simulink model "fft_direct"  (R2012b)
settings: Solver=ode45  StartTime=0.0  StopTime=199  RelTol=1e-3
libraries: xbsIndex_r4 x2893
(part 1 of 15)
settings Model: Creator=sgowda  LastModifiedBy=sgowda

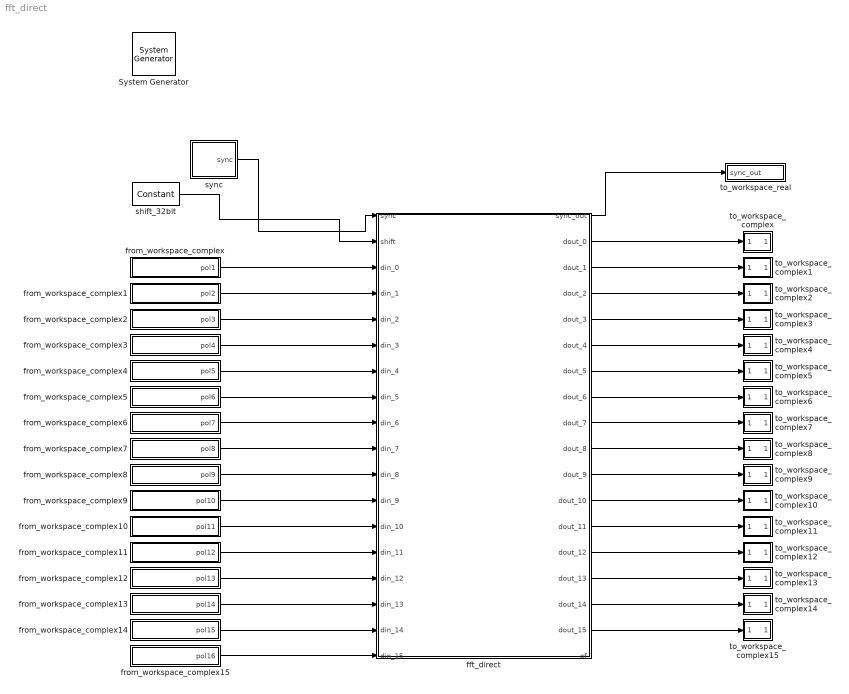
== system fft_direct ==
  " System Generator" : xbsIndex_r4/ System Generator  Tag=genX  xilinxfamily=Kintex7  part=xc7k325t  speed=-3  package=fbg676  synthesis_tool=XST  clock_wrapper=Clock Enables  directory=./netlist  proj_type=Project Navigator  Synth_file=XST Defaults  Impl_file=ISE Defaults  testbench=off  simulink_period=1  sysclk_period=10  dcm_input_clock_period=10  incr_netlist=off  trim_vbits=Everywhere in SubSystem  dbl_ovrd=According to Block Masks  core_generation=According to Block Masks  run_coregen=off  deprecated_control=off  eval_field=0  block_type=sysgen
  fft_direct : Subsystem
  from_workspace_complex : Subsystem  mask{var_name=pol1, n_bits=18, bin_pt=17, quantization=Truncate, overflow=Wrap, arith_type=Signed  (2's comp)}
      mask prompts: var_name "Workspace variable name"; n_bits "# of bits"; bin_pt "Binary Point"; arith_type "Arithmetic type"
      mask init:
      | config.source = str2func('mat_input_data_cplx_init_xblock');
      | config.toplevel = gcb();
      | xBlock(config, {config.toplevel, 'var_name', var_name, ...
      |     'n_bits', n_bits, 'bin_pt', bin_pt, 'quantization', quantization, ...
      |     'overflow', overflow, 'arith_type', arith_type});
      mask TypeOptions quantization: Truncate | Round  (unbiased: +/- Inf) | Round  (unbiased: Even Values)
      mask TypeOptions overflow: Wrap | Saturate | Flag as error
      mask TypeOptions arith_type: Signed  (2's comp) | Boolean | Unsigned
  from_workspace_complex1 : Subsystem  mask{var_name=pol2, n_bits=18, bin_pt=17, quantization=Truncate, overflow=Wrap, arith_type=Signed  (2's comp)}
      mask prompts: var_name "Workspace variable name"; n_bits "# of bits"; bin_pt "Binary Point"; arith_type "Arithmetic type"
      mask init: same as fft_direct/from_workspace_complex
      mask TypeOptions quantization: Truncate | Round  (unbiased: +/- Inf) | Round  (unbiased: Even Values)
      mask TypeOptions overflow: Wrap | Saturate | Flag as error
      mask TypeOptions arith_type: Signed  (2's comp) | Boolean | Unsigned
  from_workspace_complex10 : Subsystem  mask{var_name=pol11, n_bits=18, bin_pt=17, quantization=Truncate, overflow=Wrap, arith_type=Signed  (2's comp)}
      mask prompts: var_name "Workspace variable name"; n_bits "# of bits"; bin_pt "Binary Point"; arith_type "Arithmetic type"
      mask init: same as fft_direct/from_workspace_complex
      mask TypeOptions quantization: Truncate | Round  (unbiased: +/- Inf) | Round  (unbiased: Even Values)
      mask TypeOptions overflow: Wrap | Saturate | Flag as error
      mask TypeOptions arith_type: Signed  (2's comp) | Boolean | Unsigned
  from_workspace_complex11 : Subsystem  mask{var_name=pol12, n_bits=18, bin_pt=17, quantization=Truncate, overflow=Wrap, arith_type=Signed  (2's comp)}
      mask prompts: var_name "Workspace variable name"; n_bits "# of bits"; bin_pt "Binary Point"; arith_type "Arithmetic type"
      mask init: same as fft_direct/from_workspace_complex
      mask TypeOptions quantization: Truncate | Round  (unbiased: +/- Inf) | Round  (unbiased: Even Values)
      mask TypeOptions overflow: Wrap | Saturate | Flag as error
      mask TypeOptions arith_type: Signed  (2's comp) | Boolean | Unsigned
  from_workspace_complex12 : Subsystem  mask{var_name=pol13, n_bits=18, bin_pt=17, quantization=Truncate, overflow=Wrap, arith_type=Signed  (2's comp)}
      mask prompts: var_name "Workspace variable name"; n_bits "# of bits"; bin_pt "Binary Point"; arith_type "Arithmetic type"
      mask init: same as fft_direct/from_workspace_complex
      mask TypeOptions quantization: Truncate | Round  (unbiased: +/- Inf) | Round  (unbiased: Even Values)
      mask TypeOptions overflow: Wrap | Saturate | Flag as error
      mask TypeOptions arith_type: Signed  (2's comp) | Boolean | Unsigned
  from_workspace_complex13 : Subsystem  mask{var_name=pol14, n_bits=18, bin_pt=17, quantization=Truncate, overflow=Wrap, arith_type=Signed  (2's comp)}
      mask prompts: var_name "Workspace variable name"; n_bits "# of bits"; bin_pt "Binary Point"; arith_type "Arithmetic type"
      mask init: same as fft_direct/from_workspace_complex
      mask TypeOptions quantization: Truncate | Round  (unbiased: +/- Inf) | Round  (unbiased: Even Values)
      mask TypeOptions overflow: Wrap | Saturate | Flag as error
      mask TypeOptions arith_type: Signed  (2's comp) | Boolean | Unsigned
  from_workspace_complex14 : Subsystem  mask{var_name=pol15, n_bits=18, bin_pt=17, quantization=Truncate, overflow=Wrap, arith_type=Signed  (2's comp)}
      mask prompts: var_name "Workspace variable name"; n_bits "# of bits"; bin_pt "Binary Point"; arith_type "Arithmetic type"
      mask init: same as fft_direct/from_workspace_complex
      mask TypeOptions quantization: Truncate | Round  (unbiased: +/- Inf) | Round  (unbiased: Even Values)
      mask TypeOptions overflow: Wrap | Saturate | Flag as error
      mask TypeOptions arith_type: Signed  (2's comp) | Boolean | Unsigned
  from_workspace_complex15 : Subsystem  mask{var_name=pol16, n_bits=18, bin_pt=17, quantization=Truncate, overflow=Wrap, arith_type=Signed  (2's comp)}
      mask prompts: var_name "Workspace variable name"; n_bits "# of bits"; bin_pt "Binary Point"; arith_type "Arithmetic type"
      mask init: same as fft_direct/from_workspace_complex
      mask TypeOptions quantization: Truncate | Round  (unbiased: +/- Inf) | Round  (unbiased: Even Values)
      mask TypeOptions overflow: Wrap | Saturate | Flag as error
      mask TypeOptions arith_type: Signed  (2's comp) | Boolean | Unsigned
  from_workspace_complex2 : Subsystem  mask{var_name=pol3, n_bits=18, bin_pt=17, quantization=Truncate, overflow=Wrap, arith_type=Signed  (2's comp)}
      mask prompts: var_name "Workspace variable name"; n_bits "# of bits"; bin_pt "Binary Point"; arith_type "Arithmetic type"
      mask init: same as fft_direct/from_workspace_complex
      mask TypeOptions quantization: Truncate | Round  (unbiased: +/- Inf) | Round  (unbiased: Even Values)
      mask TypeOptions overflow: Wrap | Saturate | Flag as error
      mask TypeOptions arith_type: Signed  (2's comp) | Boolean | Unsigned
  from_workspace_complex3 : Subsystem  mask{var_name=pol4, n_bits=18, bin_pt=17, quantization=Truncate, overflow=Wrap, arith_type=Signed  (2's comp)}
      mask prompts: var_name "Workspace variable name"; n_bits "# of bits"; bin_pt "Binary Point"; arith_type "Arithmetic type"
      mask init: same as fft_direct/from_workspace_complex
      mask TypeOptions quantization: Truncate | Round  (unbiased: +/- Inf) | Round  (unbiased: Even Values)
      mask TypeOptions overflow: Wrap | Saturate | Flag as error
      mask TypeOptions arith_type: Signed  (2's comp) | Boolean | Unsigned
  from_workspace_complex4 : Subsystem  mask{var_name=pol5, n_bits=18, bin_pt=17, quantization=Truncate, overflow=Wrap, arith_type=Signed  (2's comp)}
      mask prompts: var_name "Workspace variable name"; n_bits "# of bits"; bin_pt "Binary Point"; arith_type "Arithmetic type"
      mask init: same as fft_direct/from_workspace_complex
      mask TypeOptions quantization: Truncate | Round  (unbiased: +/- Inf) | Round  (unbiased: Even Values)
      mask TypeOptions overflow: Wrap | Saturate | Flag as error
      mask TypeOptions arith_type: Signed  (2's comp) | Boolean | Unsigned
  from_workspace_complex5 : Subsystem  mask{var_name=pol6, n_bits=18, bin_pt=17, quantization=Truncate, overflow=Wrap, arith_type=Signed  (2's comp)}
      mask prompts: var_name "Workspace variable name"; n_bits "# of bits"; bin_pt "Binary Point"; arith_type "Arithmetic type"
      mask init: same as fft_direct/from_workspace_complex
      mask TypeOptions quantization: Truncate | Round  (unbiased: +/- Inf) | Round  (unbiased: Even Values)
      mask TypeOptions overflow: Wrap | Saturate | Flag as error
      mask TypeOptions arith_type: Signed  (2's comp) | Boolean | Unsigned
  from_workspace_complex6 : Subsystem  mask{var_name=pol7, n_bits=18, bin_pt=17, quantization=Truncate, overflow=Wrap, arith_type=Signed  (2's comp)}
      mask prompts: var_name "Workspace variable name"; n_bits "# of bits"; bin_pt "Binary Point"; arith_type "Arithmetic type"
      mask init: same as fft_direct/from_workspace_complex
      mask TypeOptions quantization: Truncate | Round  (unbiased: +/- Inf) | Round  (unbiased: Even Values)
      mask TypeOptions overflow: Wrap | Saturate | Flag as error
      mask TypeOptions arith_type: Signed  (2's comp) | Boolean | Unsigned
  from_workspace_complex7 : Subsystem  mask{var_name=pol8, n_bits=18, bin_pt=17, quantization=Truncate, overflow=Wrap, arith_type=Signed  (2's comp)}
      mask prompts: var_name "Workspace variable name"; n_bits "# of bits"; bin_pt "Binary Point"; arith_type "Arithmetic type"
      mask init: same as fft_direct/from_workspace_complex
      mask TypeOptions quantization: Truncate | Round  (unbiased: +/- Inf) | Round  (unbiased: Even Values)
      mask TypeOptions overflow: Wrap | Saturate | Flag as error
      mask TypeOptions arith_type: Signed  (2's comp) | Boolean | Unsigned
  from_workspace_complex8 : Subsystem  mask{var_name=pol9, n_bits=18, bin_pt=17, quantization=Truncate, overflow=Wrap, arith_type=Signed  (2's comp)}
      mask prompts: var_name "Workspace variable name"; n_bits "# of bits"; bin_pt "Binary Point"; arith_type "Arithmetic type"
      mask init: same as fft_direct/from_workspace_complex
      mask TypeOptions quantization: Truncate | Round  (unbiased: +/- Inf) | Round  (unbiased: Even Values)
      mask TypeOptions overflow: Wrap | Saturate | Flag as error
      mask TypeOptions arith_type: Signed  (2's comp) | Boolean | Unsigned
  from_workspace_complex9 : Subsystem  mask{var_name=pol10, n_bits=18, bin_pt=17, quantization=Truncate, overflow=Wrap, arith_type=Signed  (2's comp)}
      mask prompts: var_name "Workspace variable name"; n_bits "# of bits"; bin_pt "Binary Point"; arith_type "Arithmetic type"
      mask init: same as fft_direct/from_workspace_complex
      mask TypeOptions quantization: Truncate | Round  (unbiased: +/- Inf) | Round  (unbiased: Even Values)
      mask TypeOptions overflow: Wrap | Saturate | Flag as error
      mask TypeOptions arith_type: Signed  (2's comp) | Boolean | Unsigned
  shift_32bit : xbsIndex_r4/Constant  const=0  gui_display_data_type=Fixed-point  arith_type=Signed (2's comp)  n_bits=32  bin_pt=0  preci_type=Single  exp_width=8  frac_width=24  explicit_period=on  period=1  equ=P=C  opselect=C  inp2=PCIN>>17  opr=+  inp1=P  carry=CIN  dbl_ovrd=off  block_type=constant
  sync : Subsystem
  to_workspace_complex : Subsystem  mask{var_name=out1, n_bits=18, bin_pt=17}
      mask prompts: var_name "Workspace variable name"; n_bits "# of bits"; bin_pt "Binary Point"
      mask init:
      | config.source = str2func('mat_output_data_cplx_init_xblock');
      | config.toplevel = gcb();
      | xBlock(config, {config.toplevel, 'var_name', var_name, ...
      |     'n_bits', n_bits, 'bin_pt', bin_pt});
  to_workspace_complex1 : Subsystem  mask{var_name=out2, n_bits=18, bin_pt=17}
      mask prompts: var_name "Workspace variable name"; n_bits "# of bits"; bin_pt "Binary Point"
      mask init:
      | config.source = str2func('mat_output_data_cplx_init_xblock');
      | config.toplevel = gcb();
      | xBlock(config, {config.toplevel, 'var_name', var_name, ...
      |     'n_bits', n_bits, 'bin_pt', bin_pt});
  to_workspace_complex10 : Subsystem  mask{var_name=out11, n_bits=18, bin_pt=17}
      mask prompts: var_name "Workspace variable name"; n_bits "# of bits"; bin_pt "Binary Point"
      mask init:
      | config.source = str2func('mat_output_data_cplx_init_xblock');
      | config.toplevel = gcb();
      | xBlock(config, {config.toplevel, 'var_name', var_name, ...
      |     'n_bits', n_bits, 'bin_pt', bin_pt});
  to_workspace_complex11 : Subsystem  mask{var_name=out12, n_bits=18, bin_pt=17}
      mask prompts: var_name "Workspace variable name"; n_bits "# of bits"; bin_pt "Binary Point"
      mask init:
      | config.source = str2func('mat_output_data_cplx_init_xblock');
      | config.toplevel = gcb();
      | xBlock(config, {config.toplevel, 'var_name', var_name, ...
      |     'n_bits', n_bits, 'bin_pt', bin_pt});
  to_workspace_complex12 : Subsystem  mask{var_name=out13, n_bits=18, bin_pt=17}
      mask prompts: var_name "Workspace variable name"; n_bits "# of bits"; bin_pt "Binary Point"
      mask init:
      | config.source = str2func('mat_output_data_cplx_init_xblock');
      | config.toplevel = gcb();
      | xBlock(config, {config.toplevel, 'var_name', var_name, ...
      |     'n_bits', n_bits, 'bin_pt', bin_pt});
  to_workspace_complex13 : Subsystem  mask{var_name=out14, n_bits=18, bin_pt=17}
      mask prompts: var_name "Workspace variable name"; n_bits "# of bits"; bin_pt "Binary Point"
      mask init:
      | config.source = str2func('mat_output_data_cplx_init_xblock');
      | config.toplevel = gcb();
      | xBlock(config, {config.toplevel, 'var_name', var_name, ...
      |     'n_bits', n_bits, 'bin_pt', bin_pt});
  to_workspace_complex14 : Subsystem  mask{var_name=out15, n_bits=18, bin_pt=17}
      mask prompts: var_name "Workspace variable name"; n_bits "# of bits"; bin_pt "Binary Point"
      mask init:
      | config.source = str2func('mat_output_data_cplx_init_xblock');
      | config.toplevel = gcb();
      | xBlock(config, {config.toplevel, 'var_name', var_name, ...
      |     'n_bits', n_bits, 'bin_pt', bin_pt});
  to_workspace_complex15 : Subsystem  mask{var_name=out16, n_bits=18, bin_pt=17}
      mask prompts: var_name "Workspace variable name"; n_bits "# of bits"; bin_pt "Binary Point"
      mask init:
      | config.source = str2func('mat_output_data_cplx_init_xblock');
      | config.toplevel = gcb();
      | xBlock(config, {config.toplevel, 'var_name', var_name, ...
      |     'n_bits', n_bits, 'bin_pt', bin_pt});
  to_workspace_complex2 : Subsystem  mask{var_name=out3, n_bits=18, bin_pt=17}
      mask prompts: var_name "Workspace variable name"; n_bits "# of bits"; bin_pt "Binary Point"
      mask init:
      | config.source = str2func('mat_output_data_cplx_init_xblock');
      | config.toplevel = gcb();
      | xBlock(config, {config.toplevel, 'var_name', var_name, ...
      |     'n_bits', n_bits, 'bin_pt', bin_pt});
  to_workspace_complex3 : Subsystem  mask{var_name=out4, n_bits=18, bin_pt=17}
      mask prompts: var_name "Workspace variable name"; n_bits "# of bits"; bin_pt "Binary Point"
      mask init:
      | config.source = str2func('mat_output_data_cplx_init_xblock');
      | config.toplevel = gcb();
      | xBlock(config, {config.toplevel, 'var_name', var_name, ...
      |     'n_bits', n_bits, 'bin_pt', bin_pt});
  to_workspace_complex4 : Subsystem  mask{var_name=out5, n_bits=18, bin_pt=17}
      mask prompts: var_name "Workspace variable name"; n_bits "# of bits"; bin_pt "Binary Point"
      mask init:
      | config.source = str2func('mat_output_data_cplx_init_xblock');
      | config.toplevel = gcb();
      | xBlock(config, {config.toplevel, 'var_name', var_name, ...
      |     'n_bits', n_bits, 'bin_pt', bin_pt});
  to_workspace_complex5 : Subsystem  mask{var_name=out6, n_bits=18, bin_pt=17}
      mask prompts: var_name "Workspace variable name"; n_bits "# of bits"; bin_pt "Binary Point"
      mask init:
      | config.source = str2func('mat_output_data_cplx_init_xblock');
      | config.toplevel = gcb();
      | xBlock(config, {config.toplevel, 'var_name', var_name, ...
      |     'n_bits', n_bits, 'bin_pt', bin_pt});
  to_workspace_complex6 : Subsystem  mask{var_name=out7, n_bits=18, bin_pt=17}
      mask prompts: var_name "Workspace variable name"; n_bits "# of bits"; bin_pt "Binary Point"
      mask init:
      | config.source = str2func('mat_output_data_cplx_init_xblock');
      | config.toplevel = gcb();
      | xBlock(config, {config.toplevel, 'var_name', var_name, ...
      |     'n_bits', n_bits, 'bin_pt', bin_pt});
  to_workspace_complex7 : Subsystem  mask{var_name=out8, n_bits=18, bin_pt=17}
      mask prompts: var_name "Workspace variable name"; n_bits "# of bits"; bin_pt "Binary Point"
      mask init:
      | config.source = str2func('mat_output_data_cplx_init_xblock');
      | config.toplevel = gcb();
      | xBlock(config, {config.toplevel, 'var_name', var_name, ...
      |     'n_bits', n_bits, 'bin_pt', bin_pt});
  to_workspace_complex8 : Subsystem  mask{var_name=out9, n_bits=18, bin_pt=17}
      mask prompts: var_name "Workspace variable name"; n_bits "# of bits"; bin_pt "Binary Point"
      mask init:
      | config.source = str2func('mat_output_data_cplx_init_xblock');
      | config.toplevel = gcb();
      | xBlock(config, {config.toplevel, 'var_name', var_name, ...
      |     'n_bits', n_bits, 'bin_pt', bin_pt});
  to_workspace_complex9 : Subsystem  mask{var_name=out10, n_bits=18, bin_pt=17}
      mask prompts: var_name "Workspace variable name"; n_bits "# of bits"; bin_pt "Binary Point"
      mask init:
      | config.source = str2func('mat_output_data_cplx_init_xblock');
      | config.toplevel = gcb();
      | xBlock(config, {config.toplevel, 'var_name', var_name, ...
      |     'n_bits', n_bits, 'bin_pt', bin_pt});
  to_workspace_real : Subsystem  mask{var_name=sync_out}
      mask prompts: var_name "Workspace variable name"
      mask init:
      | config.source = str2func('mat_output_data_init_xblock');
      | config.toplevel = gcb();
      | xBlock(config, {config.toplevel, 'var_name', var_name});
  wires:
  shift_32bit/1 -> fft_direct/2(shift)
  sync/1(sync) -> fft_direct/1(sync)
  from_workspace_complex/1(pol1) -> fft_direct/3(din_0)
  from_workspace_complex2/1(pol3) -> fft_direct/5(din_2)
  from_workspace_complex3/1(pol4) -> fft_direct/6(din_3)
  fft_direct/1(sync_out) -> to_workspace_real/1(sync_out)
  fft_direct/2(dout_0) -> to_workspace_complex/1(out1)
  fft_direct/3(dout_1) -> to_workspace_complex1/1(out2)
  fft_direct/4(dout_2) -> to_workspace_complex2/1(out3)
  fft_direct/5(dout_3) -> to_workspace_complex3/1(out4)
  from_workspace_complex1/1(pol2) -> fft_direct/4(din_1)
  from_workspace_complex4/1(pol5) -> fft_direct/7(din_4)
  from_workspace_complex5/1(pol6) -> fft_direct/8(din_5)
  from_workspace_complex6/1(pol7) -> fft_direct/9(din_6)
  from_workspace_complex7/1(pol8) -> fft_direct/10(din_7)
  fft_direct/6(dout_4) -> to_workspace_complex4/1(out5)
  fft_direct/7(dout_5) -> to_workspace_complex5/1(out6)
  fft_direct/8(dout_6) -> to_workspace_complex6/1(out7)
  fft_direct/9(dout_7) -> to_workspace_complex7/1(out8)
  from_workspace_complex10/1(pol11) -> fft_direct/13(din_10)
  from_workspace_complex11/1(pol12) -> fft_direct/14(din_11)
  from_workspace_complex13/1(pol14) -> fft_direct/16(din_13)
  from_workspace_complex14/1(pol15) -> fft_direct/17(din_14)
  from_workspace_complex15/1(pol16) -> fft_direct/18(din_15)
  from_workspace_complex12/1(pol13) -> fft_direct/15(din_12)
  from_workspace_complex8/1(pol9) -> fft_direct/11(din_8)
  from_workspace_complex9/1(pol10) -> fft_direct/12(din_9)
  fft_direct/10(dout_8) -> to_workspace_complex8/1(out9)
  fft_direct/11(dout_9) -> to_workspace_complex9/1(out10)
  fft_direct/12(dout_10) -> to_workspace_complex10/1(out11)
  fft_direct/13(dout_11) -> to_workspace_complex11/1(out12)
  fft_direct/14(dout_12) -> to_workspace_complex12/1(out13)
  fft_direct/15(dout_13) -> to_workspace_complex13/1(out14)
  fft_direct/16(dout_14) -> to_workspace_complex14/1(out15)
  fft_direct/17(dout_15) -> to_workspace_complex15/1(out16)

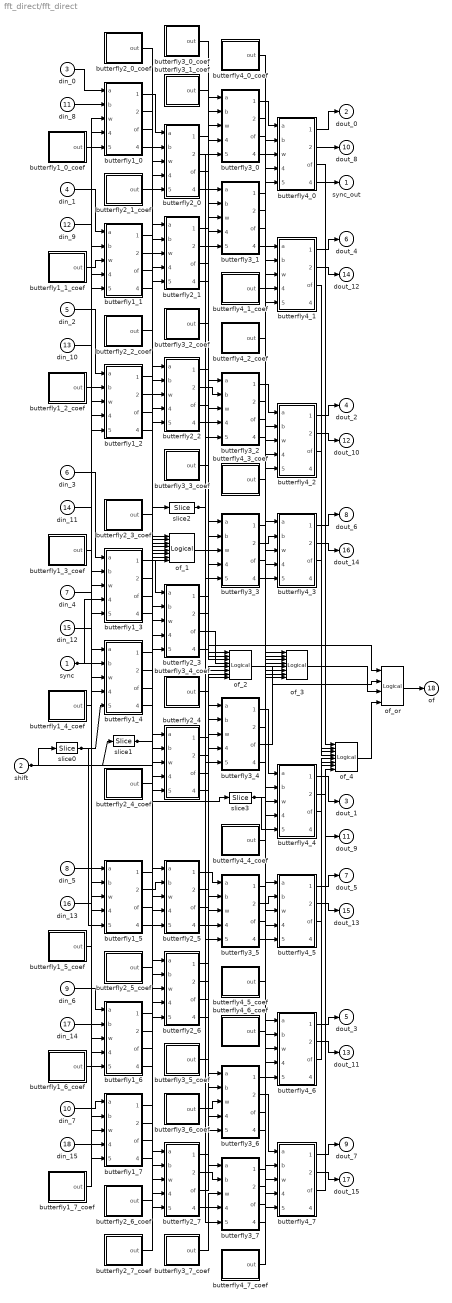
== system fft_direct/fft_direct ==
  sync : Inport
  shift : Inport  Port=2
  din_0 : Inport  Port=3
  din_1 : Inport  Port=4
  din_2 : Inport  Port=5
  din_3 : Inport  Port=6
  din_4 : Inport  Port=7
  din_5 : Inport  Port=8
  din_6 : Inport  Port=9
  din_7 : Inport  Port=10
  din_8 : Inport  Port=11
  din_9 : Inport  Port=12
  din_10 : Inport  Port=13
  din_11 : Inport  Port=14
  din_12 : Inport  Port=15
  din_13 : Inport  Port=16
  din_14 : Inport  Port=17
  din_15 : Inport  Port=18
  butterfly1_0 : Subsystem
      settings: AttributesFormatString=|
      | twiddle_pass_through
      | coeffs in slices
      | Bit growth:0
  butterfly1_0_coef : Subsystem
  butterfly1_1 : Subsystem
      settings: AttributesFormatString=|
      | twiddle_pass_through
      | coeffs in slices
      | Bit growth:0
  butterfly1_1_coef : Subsystem
  butterfly1_2 : Subsystem
      settings: AttributesFormatString=|
      | twiddle_pass_through
      | coeffs in slices
      | Bit growth:0
  butterfly1_2_coef : Subsystem
  butterfly1_3 : Subsystem
      settings: AttributesFormatString=|
      | twiddle_pass_through
      | coeffs in slices
      | Bit growth:0
  butterfly1_3_coef : Subsystem
  butterfly1_4 : Subsystem
      settings: AttributesFormatString=|
      | twiddle_pass_through
      | coeffs in slices
      | Bit growth:0
  butterfly1_4_coef : Subsystem
  butterfly1_5 : Subsystem
      settings: AttributesFormatString=|
      | twiddle_pass_through
      | coeffs in slices
      | Bit growth:0
  butterfly1_5_coef : Subsystem
  butterfly1_6 : Subsystem
      settings: AttributesFormatString=|
      | twiddle_pass_through
      | coeffs in slices
      | Bit growth:0
  butterfly1_6_coef : Subsystem
  butterfly1_7 : Subsystem
      settings: AttributesFormatString=|
      | twiddle_pass_through
      | coeffs in slices
      | Bit growth:0
  butterfly1_7_coef : Subsystem
  butterfly2_0 : Subsystem
      settings: AttributesFormatString=|
      | twiddle_pass_through
      | coeffs in slices
      | Bit growth:0
  butterfly2_0_coef : Subsystem
  butterfly2_1 : Subsystem
      settings: AttributesFormatString=|
      | twiddle_pass_through
      | coeffs in slices
      | Bit growth:0
  butterfly2_1_coef : Subsystem
  butterfly2_2 : Subsystem
      settings: AttributesFormatString=|
      | twiddle_pass_through
      | coeffs in slices
      | Bit growth:0
  butterfly2_2_coef : Subsystem
  butterfly2_3 : Subsystem
      settings: AttributesFormatString=|
      | twiddle_pass_through
      | coeffs in slices
      | Bit growth:0
  butterfly2_3_coef : Subsystem
  butterfly2_4 : Subsystem
      settings: AttributesFormatString=|
      | twiddle_coeff_1
      | coeffs in slices
      | Bit growth:0
  butterfly2_4_coef : Subsystem
  butterfly2_5 : Subsystem
      settings: AttributesFormatString=|
      | twiddle_coeff_1
      | coeffs in slices
      | Bit growth:0
  butterfly2_5_coef : Subsystem
  butterfly2_6 : Subsystem
      settings: AttributesFormatString=|
      | twiddle_coeff_1
      | coeffs in slices
      | Bit growth:0
  butterfly2_6_coef : Subsystem
  butterfly2_7 : Subsystem
      settings: AttributesFormatString=|
      | twiddle_coeff_1
      | coeffs in slices
      | Bit growth:0
  butterfly2_7_coef : Subsystem
  butterfly3_0 : Subsystem
      settings: AttributesFormatString=|
      | twiddle_general_4mult
      | coeffs in slices
      | Bit growth:0
  butterfly3_0_coef : Subsystem
  butterfly3_1 : Subsystem
      settings: AttributesFormatString=|
      | twiddle_general_4mult
      | coeffs in slices
      | Bit growth:0
  butterfly3_1_coef : Subsystem
  butterfly3_2 : Subsystem
      settings: AttributesFormatString=|
      | twiddle_general_4mult
      | coeffs in slices
      | Bit growth:0
  butterfly3_2_coef : Subsystem
  butterfly3_3 : Subsystem
      settings: AttributesFormatString=|
      | twiddle_general_4mult
      | coeffs in slices
      | Bit growth:0
  butterfly3_3_coef : Subsystem
  butterfly3_4 : Subsystem
      settings: AttributesFormatString=|
      | twiddle_general_4mult
      | coeffs in slices
      | Bit growth:0
  butterfly3_4_coef : Subsystem
  butterfly3_5 : Subsystem
      settings: AttributesFormatString=|
      | twiddle_general_4mult
      | coeffs in slices
      | Bit growth:0
  butterfly3_5_coef : Subsystem
  butterfly3_6 : Subsystem
      settings: AttributesFormatString=|
      | twiddle_general_4mult
      | coeffs in slices
      | Bit growth:0
  butterfly3_6_coef : Subsystem
  butterfly3_7 : Subsystem
      settings: AttributesFormatString=|
      | twiddle_general_4mult
      | coeffs in slices
      | Bit growth:0
  butterfly3_7_coef : Subsystem
  butterfly4_0 : Subsystem
      settings: AttributesFormatString=|
      | twiddle_general_4mult
      | coeffs in slices
      | Bit growth:0
  butterfly4_0_coef : Subsystem
  butterfly4_1 : Subsystem
      settings: AttributesFormatString=|
      | twiddle_general_4mult
      | coeffs in slices
      | Bit growth:0
  butterfly4_1_coef : Subsystem
  butterfly4_2 : Subsystem
      settings: AttributesFormatString=|
      | twiddle_general_4mult
      | coeffs in slices
      | Bit growth:0
  butterfly4_2_coef : Subsystem
  butterfly4_3 : Subsystem
      settings: AttributesFormatString=|
      | twiddle_general_4mult
      | coeffs in slices
      | Bit growth:0
  butterfly4_3_coef : Subsystem
  butterfly4_4 : Subsystem
      settings: AttributesFormatString=|
      | twiddle_general_4mult
      | coeffs in slices
      | Bit growth:0
  butterfly4_4_coef : Subsystem
  butterfly4_5 : Subsystem
      settings: AttributesFormatString=|
      | twiddle_general_4mult
      | coeffs in slices
      | Bit growth:0
  butterfly4_5_coef : Subsystem
  butterfly4_6 : Subsystem
      settings: AttributesFormatString=|
      | twiddle_general_4mult
      | coeffs in slices
      | Bit growth:0
  butterfly4_6_coef : Subsystem
  butterfly4_7 : Subsystem
      settings: AttributesFormatString=|
      | twiddle_general_4mult
      | coeffs in slices
      | Bit growth:0
  butterfly4_7_coef : Subsystem
  of_{1..4} (4 alike) : xbsIndex_r4/Logical  logical_function=OR  inputs=8  en=off  latency=1  precision=Full  arith_type=Unsigned  n_bits=16  bin_pt=0  align_bp=on  dbl_ovrd=off  block_type=logical
  of_or : xbsIndex_r4/Logical  logical_function=OR  inputs=4  en=off  latency=0  precision=Full  arith_type=Unsigned  n_bits=16  bin_pt=0  align_bp=on  dbl_ovrd=off  block_type=logical
  slice0 : xbsIndex_r4/Slice  nbits=1  boolean_output=on  mode=Lower Bit Location + Width  bit1=0  base1=MSB of Input  bit0=0  base0=LSB of Input  dbl_ovrd=off  block_type=slice
  slice1 : xbsIndex_r4/Slice  nbits=1  boolean_output=on  mode=Lower Bit Location + Width  bit1=0  base1=MSB of Input  bit0=1  base0=LSB of Input  dbl_ovrd=off  block_type=slice
  slice2 : xbsIndex_r4/Slice  nbits=1  boolean_output=on  mode=Lower Bit Location + Width  bit1=0  base1=MSB of Input  bit0=2  base0=LSB of Input  dbl_ovrd=off  block_type=slice
  slice3 : xbsIndex_r4/Slice  nbits=1  boolean_output=on  mode=Lower Bit Location + Width  bit1=0  base1=MSB of Input  bit0=3  base0=LSB of Input  dbl_ovrd=off  block_type=slice
  sync_out : Outport
  dout_0 : Outport  Port=2
  dout_1 : Outport  Port=3
  dout_2 : Outport  Port=4
  dout_3 : Outport  Port=5
  dout_4 : Outport  Port=6
  dout_5 : Outport  Port=7
  dout_6 : Outport  Port=8
  dout_7 : Outport  Port=9
  dout_8 : Outport  Port=10
  dout_9 : Outport  Port=11
  dout_10 : Outport  Port=12
  dout_11 : Outport  Port=13
  dout_12 : Outport  Port=14
  dout_13 : Outport  Port=15
  dout_14 : Outport  Port=16
  dout_15 : Outport  Port=17
  of : Outport  Port=18
  wires:
  shift/1 -> slice3/1, slice2/1, slice1/1, slice0/1
  sync/1 -> butterfly1_7/4(sync), butterfly1_6/4(sync), butterfly1_5/4(sync), butterfly1_4/4(sync), butterfly1_3/4(sync), butterfly1_2/4(sync), butterfly1_1/4(sync), butterfly1_0/4(sync)
  slice0/1 -> butterfly1_7/5(shift), butterfly1_6/5(shift), butterfly1_5/5(shift), butterfly1_4/5(shift), butterfly1_3/5(shift), butterfly1_2/5(shift), butterfly1_1/5(shift), butterfly1_0/5(shift)
  slice1/1 -> butterfly2_7/5(shift), butterfly2_6/5(shift), butterfly2_5/5(shift), butterfly2_4/5(shift), butterfly2_3/5(shift), butterfly2_2/5(shift), butterfly2_1/5(shift), butterfly2_0/5(shift)
  slice2/1 -> butterfly3_7/5(shift), butterfly3_6/5(shift), butterfly3_5/5(shift), butterfly3_4/5(shift), butterfly3_3/5(shift), butterfly3_2/5(shift), butterfly3_1/5(shift), butterfly3_0/5(shift)
  slice3/1 -> butterfly4_7/5(shift), butterfly4_6/5(shift), butterfly4_5/5(shift), butterfly4_4/5(shift), butterfly4_3/5(shift), butterfly4_2/5(shift), butterfly4_1/5(shift), butterfly4_0/5(shift)
  butterfly4_7/2(a-bw) -> dout_15/1
  butterfly4_3/2(a-bw) -> dout_14/1
  butterfly4_5/2(a-bw) -> dout_13/1
  butterfly4_1/2(a-bw) -> dout_12/1
  butterfly4_6/2(a-bw) -> dout_11/1
  butterfly4_2/2(a-bw) -> dout_10/1
  butterfly4_4/2(a-bw) -> dout_9/1
  butterfly4_0/2(a-bw) -> dout_8/1
  butterfly4_7/1(a+bw) -> dout_7/1
  butterfly4_3/1(a+bw) -> dout_6/1
  butterfly4_5/1(a+bw) -> dout_5/1
  butterfly4_1/1(a+bw) -> dout_4/1
  butterfly4_6/1(a+bw) -> dout_3/1
  butterfly4_2/1(a+bw) -> dout_2/1
  butterfly4_4/1(a+bw) -> dout_1/1
  butterfly4_0/1(a+bw) -> dout_0/1
  of_or/1 -> of/1
  of_4/1 -> of_or/4
  of_3/1 -> of_or/3
  of_2/1 -> of_or/2
  of_1/1 -> of_or/1
  butterfly4_7/3(of) -> of_4/8
  butterfly4_6/3(of) -> of_4/7
  butterfly4_5/3(of) -> of_4/6
  butterfly4_4/3(of) -> of_4/5
  butterfly4_3/3(of) -> of_4/4
  butterfly4_2/3(of) -> of_4/3
  butterfly4_1/3(of) -> of_4/2
  butterfly4_0/3(of) -> of_4/1
  butterfly3_7/4(sync_out) -> butterfly4_7/4(sync)
  butterfly4_7_coef/1(out) -> butterfly4_7/3(w)
  butterfly3_7/2(a-bw) -> butterfly4_7/2(b)
  butterfly3_6/2(a-bw) -> butterfly4_7/1(a)
  butterfly3_6/4(sync_out) -> butterfly4_6/4(sync)
  butterfly4_6_coef/1(out) -> butterfly4_6/3(w)
  butterfly3_7/1(a+bw) -> butterfly4_6/2(b)
  butterfly3_6/1(a+bw) -> butterfly4_6/1(a)
  butterfly3_5/4(sync_out) -> butterfly4_5/4(sync)
  butterfly4_5_coef/1(out) -> butterfly4_5/3(w)
  butterfly3_5/2(a-bw) -> butterfly4_5/2(b)
  butterfly3_4/2(a-bw) -> butterfly4_5/1(a)
  butterfly3_4/4(sync_out) -> butterfly4_4/4(sync)
  butterfly4_4_coef/1(out) -> butterfly4_4/3(w)
  butterfly3_5/1(a+bw) -> butterfly4_4/2(b)
  butterfly3_4/1(a+bw) -> butterfly4_4/1(a)
  butterfly3_3/4(sync_out) -> butterfly4_3/4(sync)
  butterfly4_3_coef/1(out) -> butterfly4_3/3(w)
  butterfly3_3/2(a-bw) -> butterfly4_3/2(b)
  butterfly3_2/2(a-bw) -> butterfly4_3/1(a)
  butterfly3_2/4(sync_out) -> butterfly4_2/4(sync)
  butterfly4_2_coef/1(out) -> butterfly4_2/3(w)
  butterfly3_3/1(a+bw) -> butterfly4_2/2(b)
  butterfly3_2/1(a+bw) -> butterfly4_2/1(a)
  butterfly3_1/4(sync_out) -> butterfly4_1/4(sync)
  butterfly4_1_coef/1(out) -> butterfly4_1/3(w)
  butterfly3_1/2(a-bw) -> butterfly4_1/2(b)
  butterfly3_0/2(a-bw) -> butterfly4_1/1(a)
  butterfly4_0/4(sync_out) -> sync_out/1
  butterfly3_0/4(sync_out) -> butterfly4_0/4(sync)
  butterfly4_0_coef/1(out) -> butterfly4_0/3(w)
  butterfly3_1/1(a+bw) -> butterfly4_0/2(b)
  butterfly3_0/1(a+bw) -> butterfly4_0/1(a)
  butterfly3_7/3(of) -> of_3/8
  butterfly3_6/3(of) -> of_3/7
  butterfly3_5/3(of) -> of_3/6
  butterfly3_4/3(of) -> of_3/5
  butterfly3_3/3(of) -> of_3/4
  butterfly3_2/3(of) -> of_3/3
  butterfly3_1/3(of) -> of_3/2
  butterfly3_0/3(of) -> of_3/1
  butterfly2_7/4(sync_out) -> butterfly3_7/4(sync)
  butterfly3_7_coef/1(out) -> butterfly3_7/3(w)
  butterfly2_7/2(a-bw) -> butterfly3_7/2(b)
  butterfly2_5/2(a-bw) -> butterfly3_7/1(a)
  butterfly2_6/4(sync_out) -> butterfly3_6/4(sync)
  butterfly3_6_coef/1(out) -> butterfly3_6/3(w)
  butterfly2_6/2(a-bw) -> butterfly3_6/2(b)
  butterfly2_4/2(a-bw) -> butterfly3_6/1(a)
  butterfly2_5/4(sync_out) -> butterfly3_5/4(sync)
  butterfly3_5_coef/1(out) -> butterfly3_5/3(w)
  butterfly2_7/1(a+bw) -> butterfly3_5/2(b)
  butterfly2_5/1(a+bw) -> butterfly3_5/1(a)
  butterfly2_4/4(sync_out) -> butterfly3_4/4(sync)
  butterfly3_4_coef/1(out) -> butterfly3_4/3(w)
  butterfly2_6/1(a+bw) -> butterfly3_4/2(b)
  butterfly2_4/1(a+bw) -> butterfly3_4/1(a)
  butterfly2_3/4(sync_out) -> butterfly3_3/4(sync)
  butterfly3_3_coef/1(out) -> butterfly3_3/3(w)
  butterfly2_3/2(a-bw) -> butterfly3_3/2(b)
  butterfly2_1/2(a-bw) -> butterfly3_3/1(a)
  butterfly2_2/4(sync_out) -> butterfly3_2/4(sync)
  butterfly3_2_coef/1(out) -> butterfly3_2/3(w)
  butterfly2_2/2(a-bw) -> butterfly3_2/2(b)
  butterfly2_0/2(a-bw) -> butterfly3_2/1(a)
  butterfly2_1/4(sync_out) -> butterfly3_1/4(sync)
  butterfly3_1_coef/1(out) -> butterfly3_1/3(w)
  butterfly2_3/1(a+bw) -> butterfly3_1/2(b)
  butterfly2_1/1(a+bw) -> butterfly3_1/1(a)
  butterfly2_0/4(sync_out) -> butterfly3_0/4(sync)
  butterfly3_0_coef/1(out) -> butterfly3_0/3(w)
  butterfly2_2/1(a+bw) -> butterfly3_0/2(b)
  butterfly2_0/1(a+bw) -> butterfly3_0/1(a)
  butterfly2_7/3(of) -> of_2/8
  butterfly2_6/3(of) -> of_2/7
  butterfly2_5/3(of) -> of_2/6
  butterfly2_4/3(of) -> of_2/5
  butterfly2_3/3(of) -> of_2/4
  butterfly2_2/3(of) -> of_2/3
  butterfly2_1/3(of) -> of_2/2
  butterfly2_0/3(of) -> of_2/1
  butterfly1_7/4(sync_out) -> butterfly2_7/4(sync)
  butterfly2_7_coef/1(out) -> butterfly2_7/3(w)
  butterfly1_7/2(a-bw) -> butterfly2_7/2(b)
  butterfly1_3/2(a-bw) -> butterfly2_7/1(a)
  butterfly1_6/4(sync_out) -> butterfly2_6/4(sync)
  butterfly2_6_coef/1(out) -> butterfly2_6/3(w)
  butterfly1_6/2(a-bw) -> butterfly2_6/2(b)
  butterfly1_2/2(a-bw) -> butterfly2_6/1(a)
  butterfly1_5/4(sync_out) -> butterfly2_5/4(sync)
  butterfly2_5_coef/1(out) -> butterfly2_5/3(w)
  butterfly1_5/2(a-bw) -> butterfly2_5/2(b)
  butterfly1_1/2(a-bw) -> butterfly2_5/1(a)
  butterfly1_4/4(sync_out) -> butterfly2_4/4(sync)
  butterfly2_4_coef/1(out) -> butterfly2_4/3(w)
  butterfly1_4/2(a-bw) -> butterfly2_4/2(b)
  butterfly1_0/2(a-bw) -> butterfly2_4/1(a)
  butterfly1_3/4(sync_out) -> butterfly2_3/4(sync)
  butterfly2_3_coef/1(out) -> butterfly2_3/3(w)
  butterfly1_7/1(a+bw) -> butterfly2_3/2(b)
  butterfly1_3/1(a+bw) -> butterfly2_3/1(a)
  butterfly1_2/4(sync_out) -> butterfly2_2/4(sync)
  butterfly2_2_coef/1(out) -> butterfly2_2/3(w)
  butterfly1_6/1(a+bw) -> butterfly2_2/2(b)
  butterfly1_2/1(a+bw) -> butterfly2_2/1(a)
  butterfly1_1/4(sync_out) -> butterfly2_1/4(sync)
  butterfly2_1_coef/1(out) -> butterfly2_1/3(w)
  butterfly1_5/1(a+bw) -> butterfly2_1/2(b)
  butterfly1_1/1(a+bw) -> butterfly2_1/1(a)
  butterfly1_0/4(sync_out) -> butterfly2_0/4(sync)
  butterfly2_0_coef/1(out) -> butterfly2_0/3(w)
  butterfly1_4/1(a+bw) -> butterfly2_0/2(b)
  butterfly1_0/1(a+bw) -> butterfly2_0/1(a)
  butterfly1_7/3(of) -> of_1/8
  butterfly1_6/3(of) -> of_1/7
  butterfly1_5/3(of) -> of_1/6
  butterfly1_4/3(of) -> of_1/5
  butterfly1_3/3(of) -> of_1/4
  butterfly1_2/3(of) -> of_1/3
  butterfly1_1/3(of) -> of_1/2
  butterfly1_0/3(of) -> of_1/1
  butterfly1_7_coef/1(out) -> butterfly1_7/3(w)
  din_15/1 -> butterfly1_7/2(b)
  din_7/1 -> butterfly1_7/1(a)
  butterfly1_6_coef/1(out) -> butterfly1_6/3(w)
  din_14/1 -> butterfly1_6/2(b)
  din_6/1 -> butterfly1_6/1(a)
  butterfly1_5_coef/1(out) -> butterfly1_5/3(w)
  din_13/1 -> butterfly1_5/2(b)
  din_5/1 -> butterfly1_5/1(a)
  butterfly1_4_coef/1(out) -> butterfly1_4/3(w)
  din_12/1 -> butterfly1_4/2(b)
  din_4/1 -> butterfly1_4/1(a)
  butterfly1_3_coef/1(out) -> butterfly1_3/3(w)
  din_11/1 -> butterfly1_3/2(b)
  din_3/1 -> butterfly1_3/1(a)
  butterfly1_2_coef/1(out) -> butterfly1_2/3(w)
  din_10/1 -> butterfly1_2/2(b)
  din_2/1 -> butterfly1_2/1(a)
  butterfly1_1_coef/1(out) -> butterfly1_1/3(w)
  din_9/1 -> butterfly1_1/2(b)
  din_1/1 -> butterfly1_1/1(a)
  butterfly1_0_coef/1(out) -> butterfly1_0/3(w)
  din_8/1 -> butterfly1_0/2(b)
  din_0/1 -> butterfly1_0/1(a)

== system fft_direct/from_workspace_complex ==
  c_to_ri_simulink : ComplexToRealImag
  gateway_imag : xbsIndex_r4/Gateway In  gui_display_data_type=Fixed-point  arith_type="Signed  (2's comp)"  n_bits=18  bin_pt=17  preci_type=Single  exp_width=8  frac_width=24  quantization=Truncate  overflow=Wrap  period=1  dbl_ovrd=off  timing_constraint=None  locs_specified=off  LOCs={}  UseAsADC=off  ADCChannel='1'  inherit_from_input=off  hdl_port=on  block_type=gatewayin
  gateway_real : xbsIndex_r4/Gateway In  gui_display_data_type=Fixed-point  arith_type="Signed  (2's comp)"  n_bits=18  bin_pt=17  preci_type=Single  exp_width=8  frac_width=24  quantization=Truncate  overflow=Wrap  period=1  dbl_ovrd=off  timing_constraint=None  locs_specified=off  LOCs={}  UseAsADC=off  ADCChannel='1'  inherit_from_input=off  hdl_port=on  block_type=gatewayin
  ri_to_c : Subsystem
  workspace_var : FromWorkspace  VariableName=pol1  SampleTime=0
  pol1 : Outport
  wires:
  ri_to_c/1(c) -> pol1/1
  gateway_imag/1 -> ri_to_c/2(im)
  gateway_real/1 -> ri_to_c/1(re)
  c_to_ri_simulink/2 -> gateway_imag/1
  c_to_ri_simulink/1 -> gateway_real/1
  workspace_var/1 -> c_to_ri_simulink/1

== system fft_direct/from_workspace_complex1 ==
  c_to_ri_simulink : ComplexToRealImag
  gateway_imag : xbsIndex_r4/Gateway In  gui_display_data_type=Fixed-point  arith_type="Signed  (2's comp)"  n_bits=18  bin_pt=17  preci_type=Single  exp_width=8  frac_width=24  quantization=Truncate  overflow=Wrap  period=1  dbl_ovrd=off  timing_constraint=None  locs_specified=off  LOCs={}  UseAsADC=off  ADCChannel='1'  inherit_from_input=off  hdl_port=on  block_type=gatewayin
  gateway_real : xbsIndex_r4/Gateway In  gui_display_data_type=Fixed-point  arith_type="Signed  (2's comp)"  n_bits=18  bin_pt=17  preci_type=Single  exp_width=8  frac_width=24  quantization=Truncate  overflow=Wrap  period=1  dbl_ovrd=off  timing_constraint=None  locs_specified=off  LOCs={}  UseAsADC=off  ADCChannel='1'  inherit_from_input=off  hdl_port=on  block_type=gatewayin
  ri_to_c : Subsystem
  workspace_var : FromWorkspace  VariableName=pol2  SampleTime=0
  pol2 : Outport
  wires:
  ri_to_c/1(c) -> pol2/1
  gateway_imag/1 -> ri_to_c/2(im)
  gateway_real/1 -> ri_to_c/1(re)
  c_to_ri_simulink/2 -> gateway_imag/1
  c_to_ri_simulink/1 -> gateway_real/1
  workspace_var/1 -> c_to_ri_simulink/1

== system fft_direct/from_workspace_complex10 ==
  c_to_ri_simulink : ComplexToRealImag
  gateway_imag : xbsIndex_r4/Gateway In  gui_display_data_type=Fixed-point  arith_type="Signed  (2's comp)"  n_bits=18  bin_pt=17  preci_type=Single  exp_width=8  frac_width=24  quantization=Truncate  overflow=Wrap  period=1  dbl_ovrd=off  timing_constraint=None  locs_specified=off  LOCs={}  UseAsADC=off  ADCChannel='1'  inherit_from_input=off  hdl_port=on  block_type=gatewayin
  gateway_real : xbsIndex_r4/Gateway In  gui_display_data_type=Fixed-point  arith_type="Signed  (2's comp)"  n_bits=18  bin_pt=17  preci_type=Single  exp_width=8  frac_width=24  quantization=Truncate  overflow=Wrap  period=1  dbl_ovrd=off  timing_constraint=None  locs_specified=off  LOCs={}  UseAsADC=off  ADCChannel='1'  inherit_from_input=off  hdl_port=on  block_type=gatewayin
  ri_to_c : Subsystem
  workspace_var : FromWorkspace  VariableName=pol11  SampleTime=0
  pol11 : Outport
  wires:
  ri_to_c/1(c) -> pol11/1
  gateway_imag/1 -> ri_to_c/2(im)
  gateway_real/1 -> ri_to_c/1(re)
  c_to_ri_simulink/2 -> gateway_imag/1
  c_to_ri_simulink/1 -> gateway_real/1
  workspace_var/1 -> c_to_ri_simulink/1

== system fft_direct/from_workspace_complex11 ==
  c_to_ri_simulink : ComplexToRealImag
  gateway_imag : xbsIndex_r4/Gateway In  gui_display_data_type=Fixed-point  arith_type="Signed  (2's comp)"  n_bits=18  bin_pt=17  preci_type=Single  exp_width=8  frac_width=24  quantization=Truncate  overflow=Wrap  period=1  dbl_ovrd=off  timing_constraint=None  locs_specified=off  LOCs={}  UseAsADC=off  ADCChannel='1'  inherit_from_input=off  hdl_port=on  block_type=gatewayin
  gateway_real : xbsIndex_r4/Gateway In  gui_display_data_type=Fixed-point  arith_type="Signed  (2's comp)"  n_bits=18  bin_pt=17  preci_type=Single  exp_width=8  frac_width=24  quantization=Truncate  overflow=Wrap  period=1  dbl_ovrd=off  timing_constraint=None  locs_specified=off  LOCs={}  UseAsADC=off  ADCChannel='1'  inherit_from_input=off  hdl_port=on  block_type=gatewayin
  ri_to_c : Subsystem
  workspace_var : FromWorkspace  VariableName=pol12  SampleTime=0
  pol12 : Outport
  wires:
  ri_to_c/1(c) -> pol12/1
  gateway_imag/1 -> ri_to_c/2(im)
  gateway_real/1 -> ri_to_c/1(re)
  c_to_ri_simulink/2 -> gateway_imag/1
  c_to_ri_simulink/1 -> gateway_real/1
  workspace_var/1 -> c_to_ri_simulink/1

== system fft_direct/from_workspace_complex12 ==
  c_to_ri_simulink : ComplexToRealImag
  gateway_imag : xbsIndex_r4/Gateway In  gui_display_data_type=Fixed-point  arith_type="Signed  (2's comp)"  n_bits=18  bin_pt=17  preci_type=Single  exp_width=8  frac_width=24  quantization=Truncate  overflow=Wrap  period=1  dbl_ovrd=off  timing_constraint=None  locs_specified=off  LOCs={}  UseAsADC=off  ADCChannel='1'  inherit_from_input=off  hdl_port=on  block_type=gatewayin
  gateway_real : xbsIndex_r4/Gateway In  gui_display_data_type=Fixed-point  arith_type="Signed  (2's comp)"  n_bits=18  bin_pt=17  preci_type=Single  exp_width=8  frac_width=24  quantization=Truncate  overflow=Wrap  period=1  dbl_ovrd=off  timing_constraint=None  locs_specified=off  LOCs={}  UseAsADC=off  ADCChannel='1'  inherit_from_input=off  hdl_port=on  block_type=gatewayin
  ri_to_c : Subsystem
  workspace_var : FromWorkspace  VariableName=pol13  SampleTime=0
  pol13 : Outport
  wires:
  ri_to_c/1(c) -> pol13/1
  gateway_imag/1 -> ri_to_c/2(im)
  gateway_real/1 -> ri_to_c/1(re)
  c_to_ri_simulink/2 -> gateway_imag/1
  c_to_ri_simulink/1 -> gateway_real/1
  workspace_var/1 -> c_to_ri_simulink/1

== system fft_direct/from_workspace_complex13 ==
  c_to_ri_simulink : ComplexToRealImag
  gateway_imag : xbsIndex_r4/Gateway In  gui_display_data_type=Fixed-point  arith_type="Signed  (2's comp)"  n_bits=18  bin_pt=17  preci_type=Single  exp_width=8  frac_width=24  quantization=Truncate  overflow=Wrap  period=1  dbl_ovrd=off  timing_constraint=None  locs_specified=off  LOCs={}  UseAsADC=off  ADCChannel='1'  inherit_from_input=off  hdl_port=on  block_type=gatewayin
  gateway_real : xbsIndex_r4/Gateway In  gui_display_data_type=Fixed-point  arith_type="Signed  (2's comp)"  n_bits=18  bin_pt=17  preci_type=Single  exp_width=8  frac_width=24  quantization=Truncate  overflow=Wrap  period=1  dbl_ovrd=off  timing_constraint=None  locs_specified=off  LOCs={}  UseAsADC=off  ADCChannel='1'  inherit_from_input=off  hdl_port=on  block_type=gatewayin
  ri_to_c : Subsystem
  workspace_var : FromWorkspace  VariableName=pol14  SampleTime=0
  pol14 : Outport
  wires:
  ri_to_c/1(c) -> pol14/1
  gateway_imag/1 -> ri_to_c/2(im)
  gateway_real/1 -> ri_to_c/1(re)
  c_to_ri_simulink/2 -> gateway_imag/1
  c_to_ri_simulink/1 -> gateway_real/1
  workspace_var/1 -> c_to_ri_simulink/1

== system fft_direct/from_workspace_complex14 ==
  c_to_ri_simulink : ComplexToRealImag
  gateway_imag : xbsIndex_r4/Gateway In  gui_display_data_type=Fixed-point  arith_type="Signed  (2's comp)"  n_bits=18  bin_pt=17  preci_type=Single  exp_width=8  frac_width=24  quantization=Truncate  overflow=Wrap  period=1  dbl_ovrd=off  timing_constraint=None  locs_specified=off  LOCs={}  UseAsADC=off  ADCChannel='1'  inherit_from_input=off  hdl_port=on  block_type=gatewayin
  gateway_real : xbsIndex_r4/Gateway In  gui_display_data_type=Fixed-point  arith_type="Signed  (2's comp)"  n_bits=18  bin_pt=17  preci_type=Single  exp_width=8  frac_width=24  quantization=Truncate  overflow=Wrap  period=1  dbl_ovrd=off  timing_constraint=None  locs_specified=off  LOCs={}  UseAsADC=off  ADCChannel='1'  inherit_from_input=off  hdl_port=on  block_type=gatewayin
  ri_to_c : Subsystem
  workspace_var : FromWorkspace  VariableName=pol15  SampleTime=0
  pol15 : Outport
  wires:
  ri_to_c/1(c) -> pol15/1
  gateway_imag/1 -> ri_to_c/2(im)
  gateway_real/1 -> ri_to_c/1(re)
  c_to_ri_simulink/2 -> gateway_imag/1
  c_to_ri_simulink/1 -> gateway_real/1
  workspace_var/1 -> c_to_ri_simulink/1

== system fft_direct/from_workspace_complex15 ==
  c_to_ri_simulink : ComplexToRealImag
  gateway_imag : xbsIndex_r4/Gateway In  gui_display_data_type=Fixed-point  arith_type="Signed  (2's comp)"  n_bits=18  bin_pt=17  preci_type=Single  exp_width=8  frac_width=24  quantization=Truncate  overflow=Wrap  period=1  dbl_ovrd=off  timing_constraint=None  locs_specified=off  LOCs={}  UseAsADC=off  ADCChannel='1'  inherit_from_input=off  hdl_port=on  block_type=gatewayin
  gateway_real : xbsIndex_r4/Gateway In  gui_display_data_type=Fixed-point  arith_type="Signed  (2's comp)"  n_bits=18  bin_pt=17  preci_type=Single  exp_width=8  frac_width=24  quantization=Truncate  overflow=Wrap  period=1  dbl_ovrd=off  timing_constraint=None  locs_specified=off  LOCs={}  UseAsADC=off  ADCChannel='1'  inherit_from_input=off  hdl_port=on  block_type=gatewayin
  ri_to_c : Subsystem
  workspace_var : FromWorkspace  VariableName=pol16  SampleTime=0
  pol16 : Outport
  wires:
  ri_to_c/1(c) -> pol16/1
  gateway_imag/1 -> ri_to_c/2(im)
  gateway_real/1 -> ri_to_c/1(re)
  c_to_ri_simulink/2 -> gateway_imag/1
  c_to_ri_simulink/1 -> gateway_real/1
  workspace_var/1 -> c_to_ri_simulink/1

== system fft_direct/from_workspace_complex2 ==
  c_to_ri_simulink : ComplexToRealImag
  gateway_imag : xbsIndex_r4/Gateway In  gui_display_data_type=Fixed-point  arith_type="Signed  (2's comp)"  n_bits=18  bin_pt=17  preci_type=Single  exp_width=8  frac_width=24  quantization=Truncate  overflow=Wrap  period=1  dbl_ovrd=off  timing_constraint=None  locs_specified=off  LOCs={}  UseAsADC=off  ADCChannel='1'  inherit_from_input=off  hdl_port=on  block_type=gatewayin
  gateway_real : xbsIndex_r4/Gateway In  gui_display_data_type=Fixed-point  arith_type="Signed  (2's comp)"  n_bits=18  bin_pt=17  preci_type=Single  exp_width=8  frac_width=24  quantization=Truncate  overflow=Wrap  period=1  dbl_ovrd=off  timing_constraint=None  locs_specified=off  LOCs={}  UseAsADC=off  ADCChannel='1'  inherit_from_input=off  hdl_port=on  block_type=gatewayin
  ri_to_c : Subsystem
  workspace_var : FromWorkspace  VariableName=pol3  SampleTime=0
  pol3 : Outport
  wires:
  ri_to_c/1(c) -> pol3/1
  gateway_imag/1 -> ri_to_c/2(im)
  gateway_real/1 -> ri_to_c/1(re)
  c_to_ri_simulink/2 -> gateway_imag/1
  c_to_ri_simulink/1 -> gateway_real/1
  workspace_var/1 -> c_to_ri_simulink/1

== system fft_direct/from_workspace_complex3 ==
  c_to_ri_simulink : ComplexToRealImag
  gateway_imag : xbsIndex_r4/Gateway In  gui_display_data_type=Fixed-point  arith_type="Signed  (2's comp)"  n_bits=18  bin_pt=17  preci_type=Single  exp_width=8  frac_width=24  quantization=Truncate  overflow=Wrap  period=1  dbl_ovrd=off  timing_constraint=None  locs_specified=off  LOCs={}  UseAsADC=off  ADCChannel='1'  inherit_from_input=off  hdl_port=on  block_type=gatewayin
  gateway_real : xbsIndex_r4/Gateway In  gui_display_data_type=Fixed-point  arith_type="Signed  (2's comp)"  n_bits=18  bin_pt=17  preci_type=Single  exp_width=8  frac_width=24  quantization=Truncate  overflow=Wrap  period=1  dbl_ovrd=off  timing_constraint=None  locs_specified=off  LOCs={}  UseAsADC=off  ADCChannel='1'  inherit_from_input=off  hdl_port=on  block_type=gatewayin
  ri_to_c : Subsystem
  workspace_var : FromWorkspace  VariableName=pol4  SampleTime=0
  pol4 : Outport
  wires:
  ri_to_c/1(c) -> pol4/1
  gateway_imag/1 -> ri_to_c/2(im)
  gateway_real/1 -> ri_to_c/1(re)
  c_to_ri_simulink/2 -> gateway_imag/1
  c_to_ri_simulink/1 -> gateway_real/1
  workspace_var/1 -> c_to_ri_simulink/1

== system fft_direct/from_workspace_complex4 ==
  c_to_ri_simulink : ComplexToRealImag
  gateway_imag : xbsIndex_r4/Gateway In  gui_display_data_type=Fixed-point  arith_type="Signed  (2's comp)"  n_bits=18  bin_pt=17  preci_type=Single  exp_width=8  frac_width=24  quantization=Truncate  overflow=Wrap  period=1  dbl_ovrd=off  timing_constraint=None  locs_specified=off  LOCs={}  UseAsADC=off  ADCChannel='1'  inherit_from_input=off  hdl_port=on  block_type=gatewayin
  gateway_real : xbsIndex_r4/Gateway In  gui_display_data_type=Fixed-point  arith_type="Signed  (2's comp)"  n_bits=18  bin_pt=17  preci_type=Single  exp_width=8  frac_width=24  quantization=Truncate  overflow=Wrap  period=1  dbl_ovrd=off  timing_constraint=None  locs_specified=off  LOCs={}  UseAsADC=off  ADCChannel='1'  inherit_from_input=off  hdl_port=on  block_type=gatewayin
  ri_to_c : Subsystem
  workspace_var : FromWorkspace  VariableName=pol5  SampleTime=0
  pol5 : Outport
  wires:
  ri_to_c/1(c) -> pol5/1
  gateway_imag/1 -> ri_to_c/2(im)
  gateway_real/1 -> ri_to_c/1(re)
  c_to_ri_simulink/2 -> gateway_imag/1
  c_to_ri_simulink/1 -> gateway_real/1
  workspace_var/1 -> c_to_ri_simulink/1

== system fft_direct/from_workspace_complex5 ==
  c_to_ri_simulink : ComplexToRealImag
  gateway_imag : xbsIndex_r4/Gateway In  gui_display_data_type=Fixed-point  arith_type="Signed  (2's comp)"  n_bits=18  bin_pt=17  preci_type=Single  exp_width=8  frac_width=24  quantization=Truncate  overflow=Wrap  period=1  dbl_ovrd=off  timing_constraint=None  locs_specified=off  LOCs={}  UseAsADC=off  ADCChannel='1'  inherit_from_input=off  hdl_port=on  block_type=gatewayin
  gateway_real : xbsIndex_r4/Gateway In  gui_display_data_type=Fixed-point  arith_type="Signed  (2's comp)"  n_bits=18  bin_pt=17  preci_type=Single  exp_width=8  frac_width=24  quantization=Truncate  overflow=Wrap  period=1  dbl_ovrd=off  timing_constraint=None  locs_specified=off  LOCs={}  UseAsADC=off  ADCChannel='1'  inherit_from_input=off  hdl_port=on  block_type=gatewayin
  ri_to_c : Subsystem
  workspace_var : FromWorkspace  VariableName=pol6  SampleTime=0
  pol6 : Outport
  wires:
  ri_to_c/1(c) -> pol6/1
  gateway_imag/1 -> ri_to_c/2(im)
  gateway_real/1 -> ri_to_c/1(re)
  c_to_ri_simulink/2 -> gateway_imag/1
  c_to_ri_simulink/1 -> gateway_real/1
  workspace_var/1 -> c_to_ri_simulink/1
